simulink model "IEEE_1547_fast_function"  (Simulink 9.2)
settings: Solver=ode4  StartTime=0.0  StopTime=5  FixedStep=Ts  RelTol=1e-3  EnableMultiTasking=on
PreLoadFcn:
  | Ts=40e-6;dec=1;Tend=170;Tstart=10;Nsig=10;Nbss=500;
PostLoadFcn:
  | Ts=40e-6;dec=1;Tend=170;Tstart=10;Nsig=10;Nbss=500;
InitFcn:
  | Ts=40e-6;dec=1;Tend=170;Tstart=10;Nsig=10;Nbss=500;
undefined symbols (not defined in the file or in its folder): magnitude
libraries: simulink x15, powerlib_meascontrol x15, rtlab x3, pePowerMeasurement x3, rtio_opalrt_common x2, powerlib x1
settings Model: ARTEMISmethode_block_infos=$$__separator__$$  Creator=DETLDAQ  LastModifiedBy=apabl  NumberOfSteps=10
settings DataIOCC: SignalLoggingSaveFormat=Dataset
settings OptimizationCC: BlockReduction=off  BooleanDataType=off  OptimizeBlockIOStorage=off  BufferReuse=off  GlobalBufferReuse=off  ExpressionFolding=off  LocalBlockOutputs=off  OptimizeDataStoreBuffers=off  BusAssignmentInplaceUpdate=off
settings DebuggingCC: SaveWithParameterizedLinksMsg=none  SignalResolutionControl=TryResolveAllWithWarning  MultiTaskDSMMsg=warning  MultiTaskCondExecSysMsg=none  FcnCallInpInsideContextMsg=error
settings HardwareCC: TargetBitPerPointer=64  TargetBitPerSizeT=64  TargetBitPerPtrDiffT=64  TargetLongLongMode=on  TargetIntDivRoundTo=Zero  TargetEndianess=LittleEndian  TargetWordSize=64  TargetHWDeviceType=MATLAB Host  ProdEqTarget=off
settings GRTTargetCC: CombineOutputUpdateFcns=on  GRTInterface=off
settings SimscapeCC: SimscapeNormalizeSystem=off

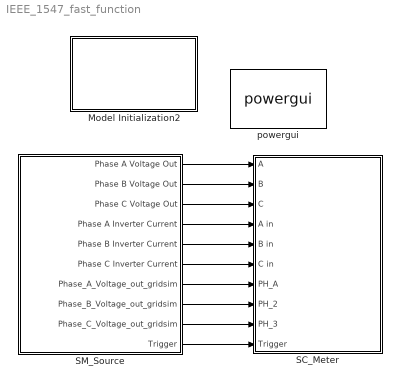
== system IEEE_1547_fast_function ==
  Model Initialization2 : Subsystem  AncestorBlock=artemis/Tools /Misc/Model Initialization  mask(Model Functions){InitFcnX=Ts=40e-6;dec=1;Tend=170;Tstart=10;Nsig=10;Nbss=500;, prel=on, posl=on, inif=on, strf=off}
      mask prompts: InitFcnX "Initialisation"; prel "Preload Function"; posl "PostLoad Function"; inif "InitFcn"; strf "StartFcn"
      mask init:
      | currentBlock = gcb;
      | root = bdroot(currentBlock);
      | 
      | if ~strcmp(get_param(root,'BlockDiagramType'),'library')
      |     if prel==1
      |         set_param(root, 'PreLoadFcn', InitFcnX);
      |     else
      |         set_param(root, 'PreLoadFcn', '');
      |     end
      |     if inif==1
      |         set_param(root, 'InitFcn', InitFcnX);
      |     else
      |         set_param(root, 'InitFcn', '');
      |     end
      |     if strf==1
      |         set_param(root, 'StartFcn', InitFcnX);
      |     else
      |         set_param(root, 'StartFcn', '');
      |     end
      |     if posl==1
      |         set_param(root, 'PostLoadFcn', InitFcnX);
      |     else
      |         set_param(root, 'PostLoadFcn', '');
      |     end
      | end
      | 
      | pos = get_param(currentBlock, 'Position');
      | width = pos(3) - pos(1); height = pos(4) - pos(2);
      | txt = [ upper(root) '\n' '- InitFcn. . . . . '  get_param(root, 'InitFcn') ];
      settings: CopyFcn=set_param(gcb,'LinkStatus','inactive')
      mask Display: text(5, height*0.5, txt, 'horizontalAlignment', 'left', 'verticalAlignment', 'middle') ;
  SC_Meter : Subsystem
  SM_Source : Subsystem
  powergui : powerlib/powergui  Priority=1  SimulationMode=Discrete  SampleTime=Ts  frequency=60  Iterations=50  frequencyindice=0  Pbase=100e6  ErrMax=1e-4  UnitsV=kV  UnitsW=MW  buscounter=0  FunctionMessages=off  echomessages=off  EnableUseOfTLC=off  CurrentSourceSwitches=off  DisableSnubberDevices=off  DisableRonSwitches=off  DisableVfSwitches=off  DisplayEquations=off  SolverType=Backward Euler  Interpol=off  ExternalGateDelay=off  methode=off  Ts=100  x0status=blocks  SPID=off  SwTol=0  HookPort=off  RestoreLinks=warning  ResistiveCurrentMeasurement=off  Frange=[0:2:500]  Ylog=off  Xlog=on  ShowGrid=off  save=off  variable=ZData  structure=0  ZoomFFT=off  StartTime=0.0  cycles=1  DisplayStyle=1  fundamental=60  FreqAxis=off  MaxFrequency=1000  frequencyindicesteady=1  RmsSteady=1  display=off
  wires:
  SM_Source/5(Phase B Inverter Current) -> SC_Meter/5(B in)
  SM_Source/6(Phase C Inverter Current) -> SC_Meter/6(C in)
  SM_Source/4(Phase A Inverter Current) -> SC_Meter/4(A in)
  SM_Source/2(Phase B Voltage Out) -> SC_Meter/2(B)
  SM_Source/1(Phase A Voltage Out) -> SC_Meter/1(A)
  SM_Source/3(Phase C Voltage Out) -> SC_Meter/3(C)
  SM_Source/7(Phase_A_Voltage_out_gridsim) -> SC_Meter/7(PH_A)
  SM_Source/8(Phase_B_Voltage_out_gridsim) -> SC_Meter/8(PH_2)
  SM_Source/9(Phase_C_Voltage_out_gridsim) -> SC_Meter/9(PH_3)
  SM_Source/10(Trigger) -> SC_Meter/10(Trigger)

== system IEEE_1547_fast_function/Model Initialization2 ==

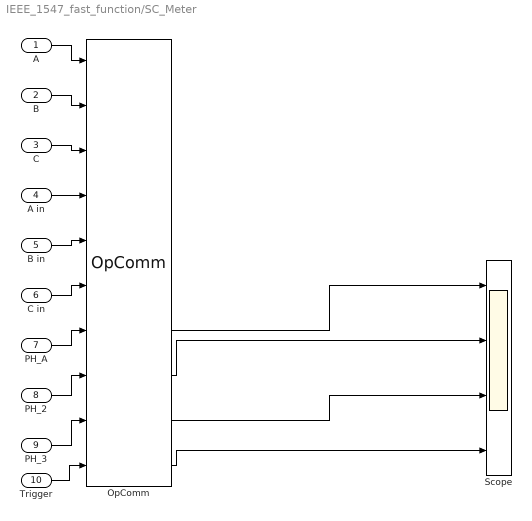
== system IEEE_1547_fast_function/SC_Meter ==
  A : Inport
  B : Inport  Port=2
  C : Inport  Port=3
  A in : Inport  Port=4
  B in : Inport  Port=5
  C in : Inport  Port=6
  PH_A : Inport  Port=7
  PH_2 : Inport  Port=8
  PH_3 : Inport  Port=9
  Trigger : Inport  Port=10
  OpComm : rtlab/OpComm  nbport=10  groupe_acq=1  subsys_rate=Ts  st=0  Synchronization=on  Interpolation=on  Threshold=1.0  Missed_Data=off  Sim_Time=off  Samples=off  dynSigOut=off  from_console=0  warning_done=off  writeOpCommFile=off  Offset=off
      settings: SourceProductName=RT-LAB
  Scope : Scope  NumInputPorts=4
  wires:
  A/1 -> OpComm/1
  B/1 -> OpComm/2
  C/1 -> OpComm/3
  A in/1 -> OpComm/4
  B in/1 -> OpComm/5
  C in/1 -> OpComm/6
  PH_A/1 -> OpComm/7
  PH_2/1 -> OpComm/8
  PH_3/1 -> OpComm/9
  Trigger/1 -> OpComm/10
  OpComm/10 -> Scope/4
  OpComm/7 -> Scope/1
  OpComm/8 -> Scope/2
  OpComm/9 -> Scope/3

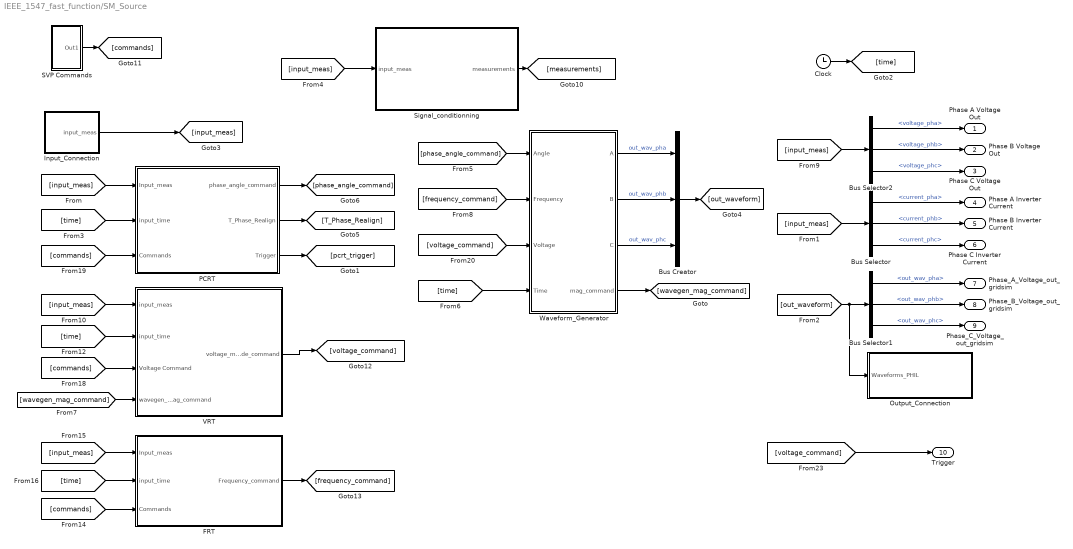
== system IEEE_1547_fast_function/SM_Source ==
  Bus Creator : BusCreator  Inputs=3
  Bus Selector : BusSelector  OutputSignals=current_pha,current_phb,current_phc
  Bus Selector1 : BusSelector  OutputSignals=out_wav_pha,out_wav_phb,out_wav_phc
  Bus Selector2 : BusSelector  OutputSignals=voltage_pha,voltage_phb,voltage_phc
  Clock : Clock
  FRT : Subsystem
  Input_Connection : Subsystem
  Output_Connection : Subsystem
  PCRT : Subsystem
  SVP Commands : Subsystem
  Signal_conditionning : Subsystem
  VRT : Subsystem
  Waveform_Generator : Subsystem
  Phase A Voltage Out : Outport
  Phase B Voltage Out : Outport  Port=2
  Phase C Voltage Out : Outport  Port=3
  Phase A Inverter Current : Outport  Port=4
  Phase B Inverter Current : Outport  Port=5
  Phase C Inverter Current : Outport  Port=6
  Phase_A_Voltage_out_gridsim : Outport  Port=7
  Phase_B_Voltage_out_gridsim : Outport  Port=8
  Phase_C_Voltage_out_gridsim : Outport  Port=9
  Trigger : Outport  Port=10
  wires:
  [frequency_command] -> Waveform_Generator/2(Frequency)
  [voltage_command] -> Waveform_Generator/3(Voltage)
  Input_Connection/1(input_meas) -> [input_meas]
  [input_meas] -> PCRT/1(Input_meas)
  [input_meas] -> Bus Selector/1
  Bus Selector/1 -> Phase A Inverter Current/1  "<current_pha>"
  Bus Selector/2 -> Phase B Inverter Current/1  "<current_phb>"
  Bus Selector/3 -> Phase C Inverter Current/1  "<current_phc>"
  Waveform_Generator/1(A) -> Bus Creator/1  "out_wav_pha"
  Waveform_Generator/2(B) -> Bus Creator/2  "out_wav_phb"
  Waveform_Generator/3(C) -> Bus Creator/3  "out_wav_phc"
  Bus Creator/1 -> [out_waveform]
  Bus Selector1/2 -> Phase_B_Voltage_out_gridsim/1  "<out_wav_phb>"
  Bus Selector1/1 -> Phase_A_Voltage_out_gridsim/1  "<out_wav_pha>"
  [out_waveform] -> Output_Connection/1(Waveforms_PHIL), Bus Selector1/1
  Bus Selector1/3 -> Phase_C_Voltage_out_gridsim/1  "<out_wav_phc>"
  PCRT/3(Trigger) -> [pcrt_trigger]
  Clock/1 -> [time]
  [time] -> PCRT/2(input_time)
  [input_meas] -> Signal_conditionning/1(input_meas)
  Signal_conditionning/1(measurements) -> [measurements]
  PCRT/2(T_Phase_Realign) -> [T_Phase_Realign]
  PCRT/1(phase_angle_command) -> [phase_angle_command]
  [phase_angle_command] -> Waveform_Generator/1(Angle)
  Bus Selector2/2 -> Phase B Voltage Out/1  "<voltage_phb>"
  Bus Selector2/1 -> Phase A Voltage Out/1  "<voltage_pha>"
  [input_meas] -> Bus Selector2/1
  Bus Selector2/3 -> Phase C Voltage Out/1  "<voltage_phc>"
  [voltage_command] -> Trigger/1
  [time] -> VRT/2(input_time)
  [input_meas] -> VRT/1(input_meas)
  [time] -> FRT/2(input_time)
  [input_meas] -> FRT/1(Input_meas)
  SVP Commands/1(Out1) -> [commands]
  [commands] -> VRT/3(Voltage Command)
  [commands] -> PCRT/3(Commands)
  VRT/1(voltage_magnitude_command) -> [voltage_command]
  [commands] -> FRT/3(Commands)
  FRT/1(Frequency_command) -> [frequency_command]
  [time] -> Waveform_Generator/4(Time)
  Waveform_Generator/4(mag_command) -> [wavegen_mag_command]
  [wavegen_mag_command] -> VRT/4(wavegen_mag_command)

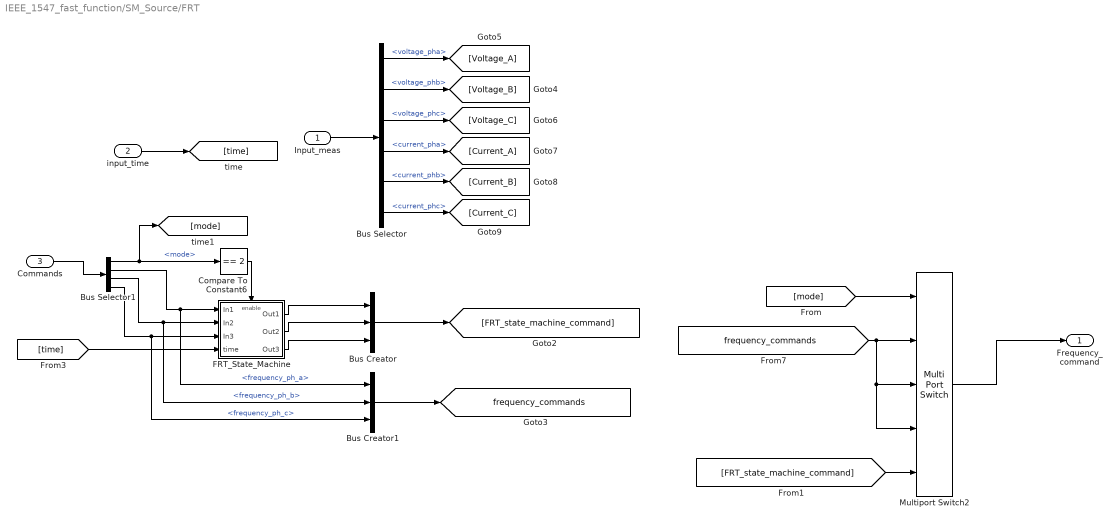
== system IEEE_1547_fast_function/SM_Source/FRT ==
  Input_meas : Inport
  input_time : Inport  Port=2
  Commands : Inport  Port=3
  Bus Creator : BusCreator  Inputs=3
  Bus Creator1 : BusCreator  Inputs=3
  Bus Selector : BusSelector  OutputSignals=voltage_pha,voltage_phb,voltage_phc,current_pha,current_phb,current_phc
  Bus Selector1 : BusSelector  OutputSignals=mode,frequency_ph_a,frequency_ph_b,frequency_ph_c
  Compare To Constant6 : simulink/Logic and Bit Operations/Compare To Constant  relop===  const=2  OutDataTypeStr=boolean
  FRT_State_Machine : Subsystem
  Multiport Switch2 : MultiPortSwitch  Inputs=4
  Frequency_command : Outport
  tag scope: frequency_commands=global
  wires:
  Input_meas/1 -> Bus Selector/1
  input_time/1 -> [time]
  FRT_State_Machine/1(Out1) -> Bus Creator/1
  FRT_State_Machine/2(Out2) -> Bus Creator/2
  FRT_State_Machine/3(Out3) -> Bus Creator/3
  Compare To Constant6/1 -> FRT_State_Machine/Enable
  Multiport Switch2/1 -> Frequency_command/1
  [mode] -> Multiport Switch2/1
  Bus Creator/1 -> [FRT_state_machine_command]
  Bus Creator1/1 -> [frequency_commands]
  [time] -> FRT_State_Machine/4(time)
  Bus Selector/1 -> [Voltage_A]  "<voltage_pha>"
  Bus Selector/2 -> [Voltage_B]  "<voltage_phb>"
  Bus Selector/3 -> [Voltage_C]  "<voltage_phc>"
  Bus Selector/4 -> [Current_A]  "<current_pha>"
  Bus Selector/5 -> [Current_B]  "<current_phb>"
  Bus Selector/6 -> [Current_C]  "<current_phc>"
  [FRT_state_machine_command] -> Multiport Switch2/5
  Commands/1 -> Bus Selector1/1
  Bus Selector1/1 -> [mode], Compare To Constant6/1  "<mode>"
  Bus Selector1/2 -> Bus Creator1/1, FRT_State_Machine/1(In1)  "<frequency_ph_a>"
  Bus Selector1/3 -> Bus Creator1/2, FRT_State_Machine/2(In2)  "<frequency_ph_b>"
  Bus Selector1/4 -> Bus Creator1/3, FRT_State_Machine/3(In3)  "<frequency_ph_c>"
  [frequency_commands] -> Multiport Switch2/3, Multiport Switch2/4, Multiport Switch2/2

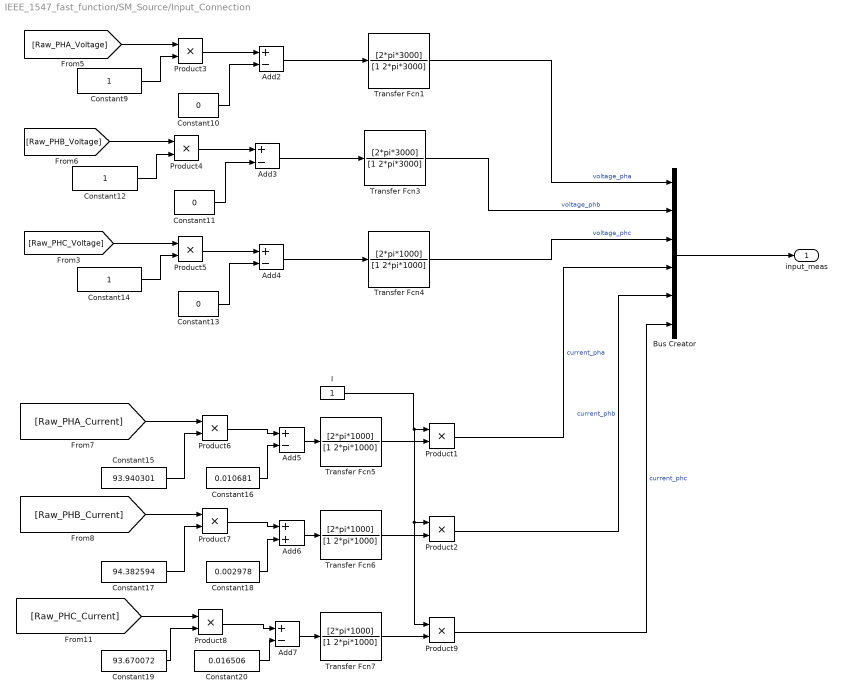
== system IEEE_1547_fast_function/SM_Source/Input_Connection ==
  Add{2..5,7} (5 alike) : Sum  Inputs=+-
  Add6 : Sum
  Bus Creator : BusCreator  Inputs=6
  Constant10 : Constant  Value=0
  Constant11 : Constant  Value=0
  Constant12 : Constant
  Constant13 : Constant  Value=0
  Constant14 : Constant
  Constant15 : Constant  Value=93.940301
  Constant16 : Constant  Value=0.010681
  Constant17 : Constant  Value=94.382594
  Constant18 : Constant  Value=0.002978
  Constant19 : Constant  Value=93.670072
  Constant20 : Constant  Value=0.016506
  Constant9 : Constant
  I : Constant
  Product{1..9} (9 alike) : Product
  Transfer Fcn1 : TransferFcn  Numerator=[2*pi*3000]  Denominator=[1 2*pi*3000]
  Transfer Fcn3 : TransferFcn  Numerator=[2*pi*3000]  Denominator=[1 2*pi*3000]
  Transfer Fcn{4..7} (4 alike) : TransferFcn  Numerator=[2*pi*1000]  Denominator=[1 2*pi*1000]
  input_meas : Outport
  wires:
  [Raw_PHB_Current] -> Product7/1
  Product6/1 -> Add5/1
  Add3/1 -> Transfer Fcn3/1
  Constant17/1 -> Product7/2
  I/1 -> Product9/1, Product2/1, Product1/1
  Transfer Fcn6/1 -> Product2/2
  Constant14/1 -> Product5/2
  Constant10/1 -> Add2/2
  Add4/1 -> Transfer Fcn4/1
  Constant13/1 -> Add4/2
  [Raw_PHB_Voltage] -> Product4/1
  Product8/1 -> Add7/1
  Product5/1 -> Add4/1
  Constant15/1 -> Product6/2
  [Raw_PHC_Voltage] -> Product5/1
  Constant20/1 -> Add7/2
  Add6/1 -> Transfer Fcn6/1
  Add5/1 -> Transfer Fcn5/1
  Product7/1 -> Add6/1
  Add2/1 -> Transfer Fcn1/1
  [Raw_PHA_Voltage] -> Product3/1
  Constant18/1 -> Add6/2
  [Raw_PHA_Current] -> Product6/1
  Transfer Fcn7/1 -> Product9/2
  [Raw_PHC_Current] -> Product8/1
  Add7/1 -> Transfer Fcn7/1
  Constant16/1 -> Add5/2
  Transfer Fcn5/1 -> Product1/2
  Constant9/1 -> Product3/2
  Constant12/1 -> Product4/2
  Product4/1 -> Add3/1
  Constant11/1 -> Add3/2
  Product3/1 -> Add2/1
  Constant19/1 -> Product8/2
  Transfer Fcn1/1 -> Bus Creator/1  "voltage_pha"
  Transfer Fcn3/1 -> Bus Creator/2  "voltage_phb"
  Transfer Fcn4/1 -> Bus Creator/3  "voltage_phc"
  Product1/1 -> Bus Creator/4  "current_pha"
  Product2/1 -> Bus Creator/5  "current_phb"
  Product9/1 -> Bus Creator/6  "current_phc"
  Bus Creator/1 -> input_meas/1

== system IEEE_1547_fast_function/SM_Source/Output_Connection ==
  Waveforms_PHIL : Inport
  AnalogOut : rtio_opalrt_common/AnalogOut  CtrlName='OpCtrl'  portNb=19  FcnNos=Slot 1 Module A Subsection 1  size=32  maxcount=-2  count=8  numchan=8  israngeinput=off  voltagerange=[-16 ... 16]  slot=0  side=0  mismatch=0  slotside=Slot_1_Module_A
      settings: AttributesFormatString=%<CtrlName>
  Bus Selector : BusSelector  OutputSignals=out_wav_pha,out_wav_phb,out_wav_phc
  Mux1 : Mux  Inputs=8
  OpCtrl : rtio_opalrt_common/OpCtrl  CtrlName='OpCtrl'  boardid=0  BitstreamFilename=VC707_2-EX-0001-3_1_6_559-eHSx128_2xC3C1FBCD-35-18.bin  numconfig=-1  mode=Master  externalClock=off  decimRtsi=0  calibIO=off  SampleTime=0  loadinport=-1  BoardType=VC707  SecondaryPresent=off  sync_type=Optical fiber  scope_enable=off  scope_acqPeriodSec=0  scope_trigPos=0
  Terminator : Terminator
  out_wav_pha : Gain
  out_wav_phb : Gain
  out_wav_phc : Gain
  wires:
  Mux1/1 -> AnalogOut/1
  AnalogOut/1 -> Terminator/1
  Waveforms_PHIL/1 -> Bus Selector/1
  Bus Selector/2 -> out_wav_phb/1  "<out_wav_phb>"
  Bus Selector/3 -> out_wav_phc/1  "<out_wav_phc>"
  Bus Selector/1 -> out_wav_pha/1  "<out_wav_pha>"
  out_wav_pha/1 -> Mux1/1
  out_wav_phb/1 -> Mux1/2
  out_wav_phc/1 -> Mux1/4

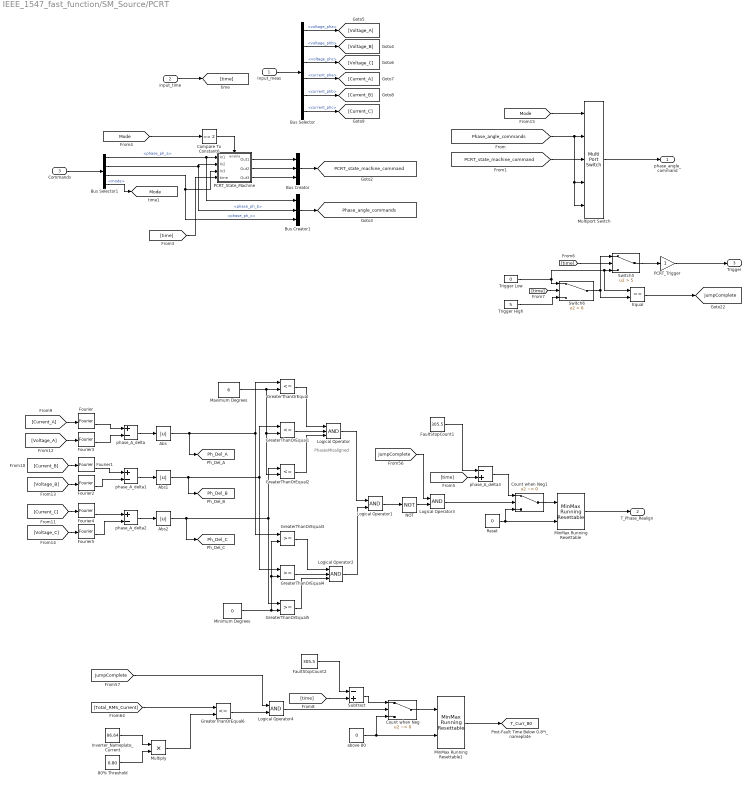
== system IEEE_1547_fast_function/SM_Source/PCRT ==
  note: PhasesMisaligned
  Input_meas : Inport
  input_time : Inport  Port=2
  Commands : Inport  Port=3
  80% Threshold : Constant  Value=0.80
  Abs : Abs
  Abs1 : Abs
  Abs2 : Abs
  Bus Creator : BusCreator  Inputs=3
  Bus Creator1 : BusCreator  Inputs=3
  Bus Selector : BusSelector  OutputSignals=voltage_pha,voltage_phb,voltage_phc,current_pha,current_phb,current_phc
  Bus Selector1 : BusSelector  OutputSignals=phase_ph_a,phase_ph_b,phase_ph_c,mode
  Compare To Constant6 : simulink/Logic and Bit Operations/Compare To Constant  relop===  const=2  OutDataTypeStr=boolean
  Count when Neg : Switch  Criteria=u2 ~= 0
  Count when Neg1 : Switch  Criteria=u2 ~= 0
  Equal : RelationalOperator  Operator===  OutDataTypeStr=boolean  RndMeth=Simplest
  FaultStopCount1 : Constant  Value=305.5
  FaultStopCount2 : Constant  Value=305.5
  Fourier{,1..5} (6 alike) : powerlib_meascontrol/Measurements/Fourier  Freq=60  n=1  InInit=[0, 0]  Ts=0
      settings: SourceProductName=Simscape Power Systems
  GreaterThanOrEqual{,1..2,6} (4 alike) : RelationalOperator  Operator=<=  OutDataTypeStr=boolean  RndMeth=Simplest
  GreaterThanOrEqual3 : RelationalOperator  OutDataTypeStr=boolean  RndMeth=Simplest
  GreaterThanOrEqual4 : RelationalOperator  OutDataTypeStr=boolean  RndMeth=Simplest
  GreaterThanOrEqual5 : RelationalOperator  OutDataTypeStr=boolean  RndMeth=Simplest
  Inverter_Nameplate_Current : Constant  Value=86.64
  Logical Operator : Logic  Inputs=3  AllPortsSameDT=off  OutDataTypeStr=boolean
  Logical Operator1 : Logic  AllPortsSameDT=off  OutDataTypeStr=boolean
  Logical Operator2 : Logic  Inputs=3  AllPortsSameDT=off  OutDataTypeStr=boolean
  Logical Operator3 : Logic  AllPortsSameDT=off  OutDataTypeStr=boolean
  Logical Operator4 : Logic  AllPortsSameDT=off  OutDataTypeStr=boolean
  Maximum Degrees : Constant  Value=6
  MinMax Running Resettable : simulink/Math Operations/MinMax Running Resettable  Function=max  vinit=0.0
  MinMax Running Resettable1 : simulink/Math Operations/MinMax Running Resettable  Function=max  vinit=0.0
  Minimum Degrees : Constant  Value=0
  Multiply : Product
  Multiport Switch : MultiPortSwitch  Inputs=4
  NOT : Logic  Operator=NOT  IconShape=distinctive  AllPortsSameDT=off  OutDataTypeStr=boolean
  PCRT_State_Machine : Subsystem
  PCRT_Trigger : Gain
  Reset : Constant  Value=0
  Subtract : Sum  Inputs=-+
  Switch5 : Switch  Criteria=u2 > Threshold  Threshold=5
  Switch6 : Switch  Criteria=u2 > Threshold  Threshold=6
  Trigger High : Constant  Value=5
  Trigger Low : Constant  Value=0
  above 80 : Constant  Value=0
  phase_A_delta : Sum  Inputs=+-
  phase_A_delta1 : Sum  Inputs=+-
  phase_A_delta2 : Sum  Inputs=+-
  phase_A_delta3 : Sum  Inputs=-+
  phase_angle_command : Outport
  T_Phase_Realign : Outport  Port=2
  Trigger : Outport  Port=3
  tag scope: JumpComplete=global, Mode=global, PCRT_state_machine_command=global, Ph_Del_A=global, Ph_Del_B=global, Ph_Del_C=global, Phase_angle_commands=global, T_Curr_80=global
  wires:
  Abs/1 -> GreaterThanOrEqual/1, GreaterThanOrEqual3/1, [Ph_Del_A]
  Abs2/1 -> GreaterThanOrEqual2/1, GreaterThanOrEqual5/1, [Ph_Del_C]
  phase_A_delta2/1 -> Abs2/1
  Abs1/1 -> GreaterThanOrEqual1/1, GreaterThanOrEqual4/1, [Ph_Del_B]
  GreaterThanOrEqual5/1 -> Logical Operator2/3
  Minimum Degrees/1 -> GreaterThanOrEqual3/2, GreaterThanOrEqual4/2, GreaterThanOrEqual5/2
  GreaterThanOrEqual/1 -> Logical Operator/1
  Reset/1 -> MinMax Running Resettable/2, Count when Neg1/3
  GreaterThanOrEqual4/1 -> Logical Operator2/2
  GreaterThanOrEqual3/1 -> Logical Operator2/1
  Logical Operator3/1 -> Count when Neg1/2
  NOT/1 -> Logical Operator3/2
  Logical Operator/1 -> Logical Operator1/1
  Fourier3/2 -> phase_A_delta/2
  Logical Operator2/1 -> Logical Operator1/2
  Logical Operator1/1 -> NOT/1
  GreaterThanOrEqual1/1 -> Logical Operator/2
  [time] -> phase_A_delta3/2
  FaultStopCount1/1 -> phase_A_delta3/1
  Maximum Degrees/1 -> GreaterThanOrEqual/2, GreaterThanOrEqual2/2, GreaterThanOrEqual1/2
  MinMax Running Resettable/1 -> T_Phase_Realign/1
  [JumpComplete] -> Logical Operator3/1
  phase_A_delta3/1 -> Count when Neg1/1
  phase_A_delta/1 -> Abs/1
  Fourier/2 -> phase_A_delta/1
  Count when Neg1/1 -> MinMax Running Resettable/1
  Fourier5/2 -> phase_A_delta2/2
  phase_A_delta1/1 -> Abs1/1
  Fourier4/2 -> phase_A_delta2/1
  GreaterThanOrEqual2/1 -> Logical Operator/3
  Fourier1/2 -> phase_A_delta1/1
  Fourier2/2 -> phase_A_delta1/2
  Input_meas/1 -> Bus Selector/1
  Trigger High/1 -> Switch6/3
  Equal/1 -> [JumpComplete]
  [time] -> Switch6/2
  Trigger Low/1 -> Equal/1, Switch5/3, Switch6/1
  PCRT_Trigger/1 -> Trigger/1
  Switch6/1 -> Equal/2, Switch5/1
  [time] -> Switch5/2
  Switch5/1 -> PCRT_Trigger/1
  input_time/1 -> [time]
  [time] -> Subtract/2
  FaultStopCount2/1 -> Subtract/1
  [JumpComplete] -> Logical Operator4/1
  Subtract/1 -> Count when Neg/1
  Multiply/1 -> GreaterThanOrEqual6/2
  Count when Neg/1 -> MinMax Running Resettable1/1
  above 80/1 -> Count when Neg/3, MinMax Running Resettable1/2
  Inverter_Nameplate_Current/1 -> Multiply/1
  [Total_RMS_Current] -> GreaterThanOrEqual6/1
  Logical Operator4/1 -> Count when Neg/2
  GreaterThanOrEqual6/1 -> Logical Operator4/2
  MinMax Running Resettable1/1 -> [T_Curr_80]
  80% Threshold/1 -> Multiply/2
  Bus Selector1/2 -> Bus Creator1/2, PCRT_State_Machine/2(In2)  "<phase_ph_b>"
  Bus Selector1/3 -> Bus Creator1/3, PCRT_State_Machine/3(In3)  "<phase_ph_c>"
  PCRT_State_Machine/1(Out1) -> Bus Creator/1
  PCRT_State_Machine/2(Out2) -> Bus Creator/2
  PCRT_State_Machine/3(Out3) -> Bus Creator/3
  Compare To Constant6/1 -> PCRT_State_Machine/Enable
  Multiport Switch/1 -> phase_angle_command/1
  [Mode] -> Multiport Switch/1
  Bus Creator/1 -> [PCRT_state_machine_command]
  Bus Creator1/1 -> [Phase_angle_commands]
  [time] -> PCRT_State_Machine/4(time)
  [Mode] -> Compare To Constant6/1
  Bus Selector/1 -> [Voltage_A]  "<voltage_pha>"
  Bus Selector/2 -> [Voltage_B]  "<voltage_phb>"
  Bus Selector/3 -> [Voltage_C]  "<voltage_phc>"
  Bus Selector/4 -> [Current_A]  "<current_pha>"
  Bus Selector/5 -> [Current_B]  "<current_phb>"
  Bus Selector/6 -> [Current_C]  "<current_phc>"
  [Current_A] -> Fourier/1
  [Current_C] -> Fourier4/1
  [Current_B] -> Fourier1/1
  [Voltage_A] -> Fourier3/1
  [Voltage_B] -> Fourier2/1
  [Voltage_C] -> Fourier5/1
  Commands/1 -> Bus Selector1/1
  Bus Selector1/1 -> Bus Creator1/1, PCRT_State_Machine/1(In1)  "<phase_ph_a>"
  Bus Selector1/4 -> [Mode]  "<mode>"
  [PCRT_state_machine_command] -> Multiport Switch/3
  [Phase_angle_commands] -> Multiport Switch/5, Multiport Switch/4, Multiport Switch/2

== system IEEE_1547_fast_function/SM_Source/SVP Commands ==
  note: Mode :
      |
      | Nothing
      | 1
      |
      | PCRT
      | 2
      |
      | VRT
      | 3
      |
      | FRT
      | 4
  Bus Creator : BusCreator  Inputs=10
  frequency_ph_a : Constant  Value=60
  frequency_ph_b : Constant  Value=60
  frequency_ph_c : Constant  Value=60
  mode : Constant  Value=3
  phase_ph_a : Constant  Value=0
  phase_ph_b : Constant  Value=-120
  phase_ph_c : Constant  Value=120
  voltage_ph_a : Constant
  voltage_ph_b : Constant
  voltage_ph_c : Constant
  Out1 : Outport
  wires:
  phase_ph_b/1 -> Bus Creator/2  "phase_ph_b"
  phase_ph_c/1 -> Bus Creator/3  "phase_ph_c"
  phase_ph_a/1 -> Bus Creator/1  "phase_ph_a"
  voltage_ph_a/1 -> Bus Creator/4  "voltage_ph_a"
  voltage_ph_c/1 -> Bus Creator/6  "voltage_ph_c"
  voltage_ph_b/1 -> Bus Creator/5  "voltage_ph_b"
  frequency_ph_b/1 -> Bus Creator/8  "frequency_ph_b"
  frequency_ph_c/1 -> Bus Creator/9  "frequency_ph_c"
  frequency_ph_a/1 -> Bus Creator/7  "frequency_ph_a"
  mode/1 -> Bus Creator/10  "mode"
  Bus Creator/1 -> Out1/1

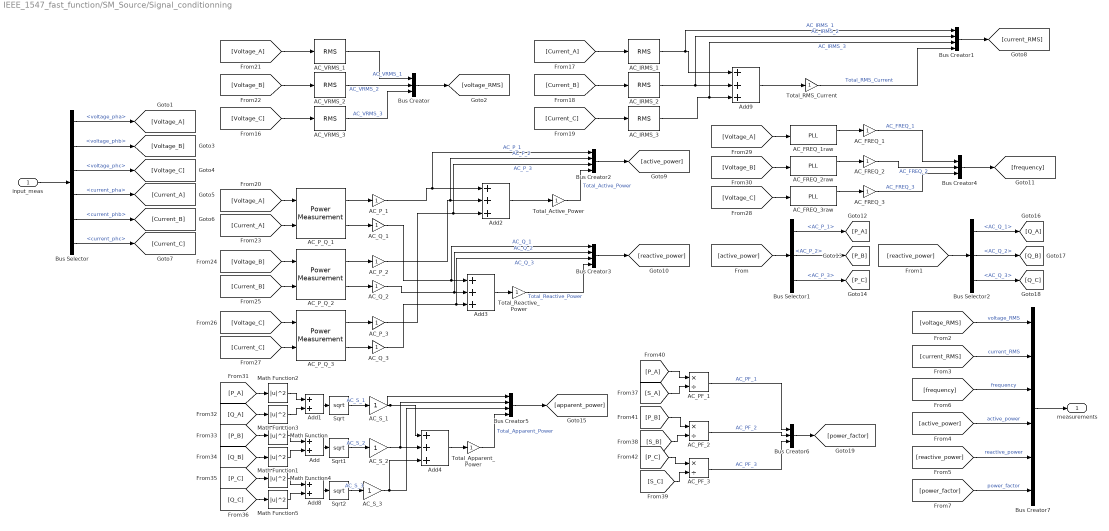
== system IEEE_1547_fast_function/SM_Source/Signal_conditionning ==
  input_meas : Inport
  AC_FREQ_1 : Gain
  AC_FREQ_1raw : powerlib_meascontrol/PLL/PLL  Fmin=45  Par_Init=[0, 60]  ParK=[180, 3200, 1]  TcD=1e-4  MaxRateChangeFreq=12  FilterCutOffFreq=25  Ts=0  AGC=on
      settings: SourceProductName=Simscape Power Systems  SourceProductBaseCode=PS
  AC_FREQ_2 : Gain
  AC_FREQ_2raw : powerlib_meascontrol/PLL/PLL  Fmin=45  Par_Init=[0, 60]  ParK=[180, 3200, 1]  TcD=1e-4  MaxRateChangeFreq=12  FilterCutOffFreq=25  Ts=0  AGC=on
      settings: SourceProductName=Simscape Power Systems  SourceProductBaseCode=PS
  AC_FREQ_3 : Gain
  AC_FREQ_3raw : powerlib_meascontrol/PLL/PLL  Fmin=45  Par_Init=[0, 60]  ParK=[180, 3200, 1]  TcD=1e-4  MaxRateChangeFreq=12  FilterCutOffFreq=25  Ts=0  AGC=on
      settings: SourceProductName=Simscape Power Systems  SourceProductBaseCode=PS
  AC_IRMS_1 : powerlib_meascontrol/Measurements/RMS  TrueRMS=on  Freq=60  RMSInit=120  Ts=0
  AC_IRMS_2 : powerlib_meascontrol/Measurements/RMS  TrueRMS=on  Freq=60  RMSInit=120  Ts=0
  AC_IRMS_3 : powerlib_meascontrol/Measurements/RMS  TrueRMS=on  Freq=60  RMSInit=120  Ts=0
  AC_PF_1 : Product  Inputs=*/
  AC_PF_2 : Product  Inputs=*/
  AC_PF_3 : Product  Inputs=*/
  AC_P_1 : Gain
  AC_P_2 : Gain
  AC_P_3 : Gain
  AC_P_Q_1 : pePowerMeasurement/Power Measurement  LabelModeActiveChoice=Continuous  F=60  K=[0 1 2 3]  Ts=0
  AC_P_Q_2 : pePowerMeasurement/Power Measurement  LabelModeActiveChoice=Continuous  F=60  K=[0 1 2 3]  Ts=0
  AC_P_Q_3 : pePowerMeasurement/Power Measurement  LabelModeActiveChoice=Continuous  F=60  K=[0 1 2 3]  Ts=0
  AC_Q_1 : Gain
  AC_Q_2 : Gain
  AC_Q_3 : Gain
  AC_S_1 : Gain
  AC_S_2 : Gain
  AC_S_3 : Gain
  AC_VRMS_1 : powerlib_meascontrol/Measurements/RMS  TrueRMS=on  Freq=60  RMSInit=120  Ts=0
  AC_VRMS_2 : powerlib_meascontrol/Measurements/RMS  TrueRMS=on  Freq=60  RMSInit=120  Ts=0
  AC_VRMS_3 : powerlib_meascontrol/Measurements/RMS  TrueRMS=on  Freq=60  RMSInit=120  Ts=0
  Add : Sum
  Add1 : Sum
  Add{2..4,9} (4 alike) : Sum  Inputs=+++
  Add8 : Sum
  Bus Creator : BusCreator  Inputs=3
  Bus Creator{1..3,5} (4 alike) : BusCreator  Inputs=4
  Bus Creator4 : BusCreator  Inputs=3
  Bus Creator6 : BusCreator  Inputs=3
  Bus Creator7 : BusCreator  Inputs=6
  Bus Selector : BusSelector  OutputSignals=voltage_pha,voltage_phb,voltage_phc,current_pha,current_phb,current_phc
  Bus Selector1 : BusSelector  OutputSignals=AC_P_1,AC_P_2,AC_P_3
  Bus Selector2 : BusSelector  OutputSignals=AC_Q_1,AC_Q_2,AC_Q_3
  Math Function{,1..5} (6 alike) : Math  Operator=magnitude^2  SaturateOnIntegerOverflow=on
  Sqrt : Sqrt  SaturateOnIntegerOverflow=on
  Sqrt1 : Sqrt  SaturateOnIntegerOverflow=on
  Sqrt2 : Sqrt  SaturateOnIntegerOverflow=on
  Total_Active_Power : Gain
  Total_Apparent_Power : Gain
  Total_RMS_Current : Gain
  Total_Reactive_Power : Gain
  measurements : Outport
  wires:
  [Current_B] -> AC_IRMS_2/1
  [P_A] -> AC_PF_1/1
  Math Function4/1 -> Add8/1
  [Voltage_A] -> AC_P_Q_1/1
  [Current_C] -> AC_IRMS_3/1
  [Current_A] -> AC_P_Q_1/2
  [Voltage_C] -> AC_VRMS_3/1
  Sqrt1/1 -> AC_S_2/1  "AC_S_2"
  [Voltage_B] -> AC_VRMS_2/1
  Math Function1/1 -> Add/2
  AC_P_Q_1/2 -> AC_Q_1/1
  Math Function5/1 -> Add8/2
  [Voltage_B] -> AC_P_Q_2/1
  [Current_A] -> AC_IRMS_1/1
  AC_P_Q_1/1 -> AC_P_1/1
  [Voltage_C] -> AC_P_Q_3/1
  AC_P_Q_2/2 -> AC_Q_2/1
  Add8/1 -> Sqrt2/1
  AC_P_Q_3/1 -> AC_P_3/1
  [Current_B] -> AC_P_Q_2/2
  [Voltage_A] -> AC_FREQ_1raw/1
  [Q_B] -> Math Function1/1
  [Voltage_C] -> AC_FREQ_3raw/1
  [P_C] -> AC_PF_3/1
  AC_FREQ_1raw/1 -> AC_FREQ_1/1
  [S_C] -> AC_PF_3/2
  [P_B] -> Math Function/1
  AC_FREQ_2raw/1 -> AC_FREQ_2/1
  [P_B] -> AC_PF_2/1
  [Q_A] -> Math Function3/1
  [Voltage_B] -> AC_FREQ_2raw/1
  Sqrt/1 -> AC_S_1/1  "AC_S_1"
  Sqrt2/1 -> AC_S_3/1  "AC_S_3"
  [P_A] -> Math Function2/1
  Add9/1 -> Total_RMS_Current/1
  Math Function3/1 -> Add1/2
  Add1/1 -> Sqrt/1
  Math Function/1 -> Add/1
  [S_B] -> AC_PF_2/2
  [Voltage_A] -> AC_VRMS_1/1
  AC_P_Q_3/2 -> AC_Q_3/1
  Math Function2/1 -> Add1/1
  [Current_C] -> AC_P_Q_3/2
  [P_C] -> Math Function4/1
  [Q_C] -> Math Function5/1
  Add/1 -> Sqrt1/1
  AC_FREQ_3raw/1 -> AC_FREQ_3/1
  AC_P_Q_2/1 -> AC_P_2/1
  [S_A] -> AC_PF_1/2
  input_meas/1 -> Bus Selector/1
  Bus Selector/1 -> [Voltage_A]  "<voltage_pha>"
  Bus Selector/2 -> [Voltage_B]  "<voltage_phb>"
  Bus Selector/3 -> [Voltage_C]  "<voltage_phc>"
  Bus Selector/4 -> [Current_A]  "<current_pha>"
  Bus Selector/5 -> [Current_B]  "<current_phb>"
  Bus Selector/6 -> [Current_C]  "<current_phc>"
  AC_P_1/1 -> Bus Creator2/1, Add2/1  "AC_P_1"
  AC_P_2/1 -> Bus Creator2/2, Add2/2  "AC_P_2"
  AC_P_3/1 -> Bus Creator2/3, Add2/3  "AC_P_3"
  Add2/1 -> Total_Active_Power/1
  AC_Q_1/1 -> Bus Creator3/1, Add3/1  "AC_Q_1"
  AC_Q_2/1 -> Bus Creator3/2, Add3/2  "AC_Q_2"
  AC_Q_3/1 -> Bus Creator3/3, Add3/3  "AC_Q_3"
  Add3/1 -> Total_Reactive_Power/1
  Add4/1 -> Total_Apparent_Power/1
  AC_VRMS_1/1 -> Bus Creator/1  "AC_VRMS_1"
  AC_VRMS_2/1 -> Bus Creator/2  "AC_VRMS_2"
  AC_VRMS_3/1 -> Bus Creator/3  "AC_VRMS_3"
  Bus Creator/1 -> [voltage_RMS]
  AC_IRMS_1/1 -> Bus Creator1/1, Add9/1  "AC_IRMS_1"
  AC_IRMS_2/1 -> Bus Creator1/2, Add9/2  "AC_IRMS_2"
  Bus Creator1/1 -> [current_RMS]
  AC_IRMS_3/1 -> Bus Creator1/3, Add9/3  "AC_IRMS_3"
  Total_RMS_Current/1 -> Bus Creator1/4  "Total_RMS_Current"
  Total_Active_Power/1 -> Bus Creator2/4  "Total_Active_Power"
  Bus Creator2/1 -> [active_power]
  Bus Creator3/1 -> [reactive_power]
  Total_Reactive_Power/1 -> Bus Creator3/4  "Total_Reactive_Power"
  Bus Creator4/1 -> [frequency]
  AC_FREQ_1/1 -> Bus Creator4/1  "AC_FREQ_1"
  AC_FREQ_2/1 -> Bus Creator4/2  "AC_FREQ_2"
  AC_FREQ_3/1 -> Bus Creator4/3  "AC_FREQ_3"
  [active_power] -> Bus Selector1/1
  Bus Selector1/1 -> [P_A]  "<AC_P_1>"
  Bus Selector1/2 -> [P_B]  "<AC_P_2>"
  Bus Selector1/3 -> [P_C]  "<AC_P_3>"
  [reactive_power] -> Bus Selector2/1
  Bus Creator5/1 -> [apparent_power]
  Total_Apparent_Power/1 -> Bus Creator5/4  "Total_Apparent_Power"
  Bus Selector2/1 -> [Q_A]  "<AC_Q_1>"
  Bus Selector2/2 -> [Q_B]  "<AC_Q_2>"
  Bus Selector2/3 -> [Q_C]  "<AC_Q_3>"
  Bus Creator6/1 -> [power_factor]
  AC_PF_3/1 -> Bus Creator6/3  "AC_PF_3"
  AC_PF_1/1 -> Bus Creator6/1  "AC_PF_1"
  AC_PF_2/1 -> Bus Creator6/2  "AC_PF_2"
  [voltage_RMS] -> Bus Creator7/1  "voltage_RMS"
  [current_RMS] -> Bus Creator7/2  "current_RMS"
  [frequency] -> Bus Creator7/3  "frequency"
  [active_power] -> Bus Creator7/4  "active_power"
  [reactive_power] -> Bus Creator7/5  "reactive_power"
  [power_factor] -> Bus Creator7/6  "power_factor"
  Bus Creator7/1 -> measurements/1
  AC_S_1/1 -> Bus Creator5/1, Add4/1
  AC_S_2/1 -> Bus Creator5/2, Add4/2
  AC_S_3/1 -> Bus Creator5/3, Add4/3

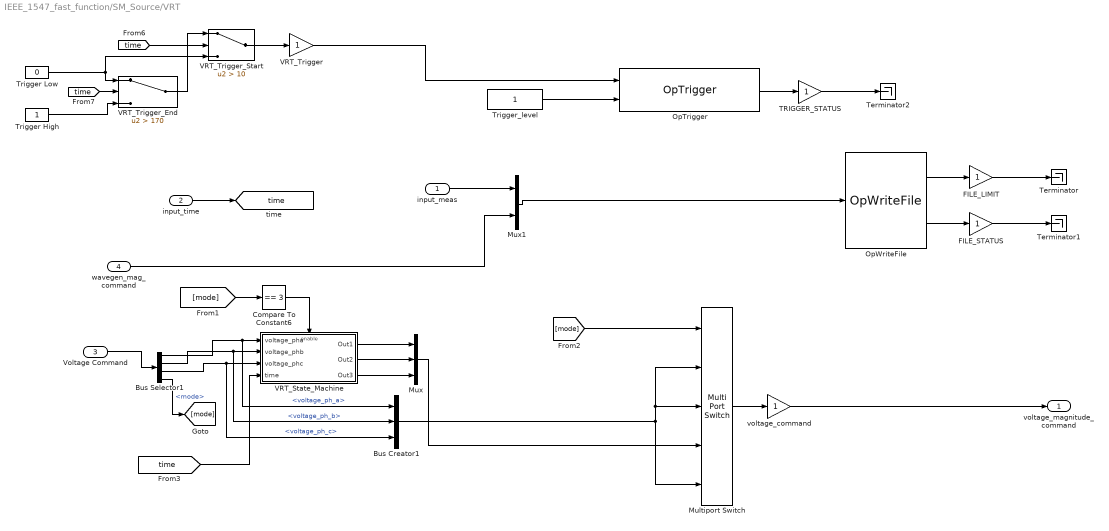
== system IEEE_1547_fast_function/SM_Source/VRT ==
  input_meas : Inport
  input_time : Inport  Port=2
  Voltage Command : Inport  Port=3
  wavegen_mag_command : Inport  Port=4
  Bus Creator1 : BusCreator  Inputs=3
  Bus Selector1 : BusSelector  OutputSignals=voltage_ph_a,voltage_ph_b,voltage_ph_c,mode
  Compare To Constant6 : simulink/Logic and Bit Operations/Compare To Constant  relop===  const=3  OutDataTypeStr=uint8
  FILE_LIMIT : Gain
  FILE_STATUS : Gain
  Multiport Switch : MultiPortSwitch  Inputs=4
  Mux : Mux  Inputs=3
  Mux1 : Mux  Inputs=2
  OpTrigger : rtlab/DataLogging/OpTrigger  Trig_Type=TRIGGER SIGNAL >= TRIGGER LEVEL  Trig_Offset=0  Acq_Group=26
      settings: SourceProductName=RT-LAB
  OpWriteFile : rtlab/DataLogging/OpWriteFile  Static_File=on  varname=Data  Filename=VRT_Data.mat  rtpath='./'  nrtpath='.\'  Acq_Group=26  file_size=2e+9  write_offline=off  Sim_Mode=off  Nb_Samples=1000  Buffer_size=88000000
      settings: SourceProductName=RT-LAB  Decimation=5
  TRIGGER_STATUS : Gain
  Terminator : Terminator
  Terminator1 : Terminator
  Terminator2 : Terminator
  Trigger High : Constant
  Trigger Low : Constant  Value=0
  Trigger_level : Constant
  VRT_State_Machine : Subsystem
  VRT_Trigger : Gain
  VRT_Trigger_End : Switch  Criteria=u2 > Threshold  Threshold=170
  VRT_Trigger_Start : Switch  Criteria=u2 > Threshold  Threshold=10
  voltage_command : Gain
  voltage_magnitude_command : Outport
  tag scope: time=global
  wires:
  [mode] -> Compare To Constant6/1
  [time] -> VRT_State_Machine/4(time)
  [mode] -> Multiport Switch/1
  Bus Creator1/1 -> Multiport Switch/2, Multiport Switch/3, Multiport Switch/5
  Compare To Constant6/1 -> VRT_State_Machine/Enable
  VRT_State_Machine/3(Out3) -> Mux/3
  VRT_State_Machine/2(Out2) -> Mux/2
  VRT_State_Machine/1(Out1) -> Mux/1
  input_time/1 -> [time]
  Voltage Command/1 -> Bus Selector1/1
  Bus Selector1/1 -> Bus Creator1/1, VRT_State_Machine/1(voltage_pha)  "<voltage_ph_a>"
  Bus Selector1/2 -> Bus Creator1/2, VRT_State_Machine/2(voltage_phb)  "<voltage_ph_b>"
  Bus Selector1/3 -> Bus Creator1/3, VRT_State_Machine/3(voltage_phc)  "<voltage_ph_c>"
  Bus Selector1/4 -> [mode]  "<mode>"
  Mux/1 -> Multiport Switch/4
  Multiport Switch/1 -> voltage_command/1
  voltage_command/1 -> voltage_magnitude_command/1
  OpWriteFile/1 -> FILE_LIMIT/1
  FILE_LIMIT/1 -> Terminator/1
  OpWriteFile/2 -> FILE_STATUS/1
  FILE_STATUS/1 -> Terminator1/1
  TRIGGER_STATUS/1 -> Terminator2/1
  Trigger_level/1 -> OpTrigger/2
  OpTrigger/1 -> TRIGGER_STATUS/1
  Mux1/1 -> OpWriteFile/1
  VRT_Trigger_End/1 -> VRT_Trigger_Start/1
  [time] -> VRT_Trigger_End/2
  Trigger High/1 -> VRT_Trigger_End/3
  VRT_Trigger/1 -> OpTrigger/1
  [time] -> VRT_Trigger_Start/2
  Trigger Low/1 -> VRT_Trigger_Start/3, VRT_Trigger_End/1
  VRT_Trigger_Start/1 -> VRT_Trigger/1
  input_meas/1 -> Mux1/1
  wavegen_mag_command/1 -> Mux1/2

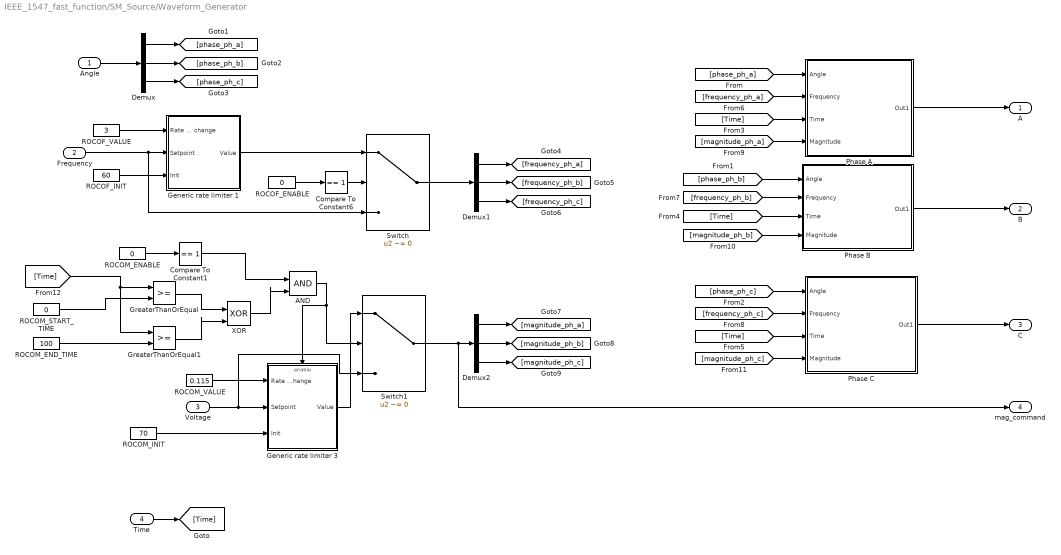
== system IEEE_1547_fast_function/SM_Source/Waveform_Generator ==
  Angle : Inport
  Frequency : Inport  Port=2
  Voltage : Inport  Port=3
  Time : Inport  Port=4
  AND : Logic  IconShape=distinctive  AllPortsSameDT=off  OutDataTypeStr=boolean
  Compare To Constant1 : simulink/Logic and Bit Operations/Compare To Constant  relop===  const=1  OutDataTypeStr=boolean
  Compare To Constant6 : simulink/Logic and Bit Operations/Compare To Constant  relop===  const=1  OutDataTypeStr=boolean
  Demux : Demux  Outputs=3
  Demux1 : Demux  Outputs=3
  Demux2 : Demux  Outputs=3
  Generic rate limiter 1 : Subsystem
  Generic rate limiter 3 : Subsystem
  GreaterThanOrEqual : RelationalOperator  OutDataTypeStr=boolean  RndMeth=Simplest
  GreaterThanOrEqual1 : RelationalOperator  OutDataTypeStr=boolean  RndMeth=Simplest
  Phase A : Subsystem
  Phase B : Subsystem
  Phase C : Subsystem
  ROCOF_ENABLE : Constant  Value=0
  ROCOF_INIT : Constant  Value=60
  ROCOF_VALUE : Constant  Value=3
  ROCOM_ENABLE : Constant  Value=0
  ROCOM_END_TIME : Constant  Value=100
  ROCOM_INIT : Constant  Value=70
  ROCOM_START_TIME : Constant  Value=0
  ROCOM_VALUE : Constant  Value=0.115
  Switch : Switch  Criteria=u2 ~= 0
  Switch1 : Switch  Criteria=u2 ~= 0
  XOR : Logic  Operator=XOR  IconShape=distinctive  AllPortsSameDT=off  OutDataTypeStr=boolean
  A : Outport
  B : Outport  Port=2
  C : Outport  Port=3
  mag_command : Outport  Port=4
  wires:
  Time/1 -> [Time]
  Phase A/1(Out1) -> A/1
  Phase B/1(Out1) -> B/1
  Phase C/1(Out1) -> C/1
  Voltage/1 -> Switch1/3, Generic rate limiter 3/2("Setpoint ")
  Angle/1 -> Demux/1
  Demux/1 -> [phase_ph_a]
  Demux/2 -> [phase_ph_b]
  Demux/3 -> [phase_ph_c]
  [phase_ph_a] -> Phase A/1(Angle)
  [phase_ph_b] -> Phase B/1(Angle)
  [phase_ph_c] -> Phase C/1(Angle)
  Generic rate limiter 1/1(Value) -> Switch/1
  Frequency/1 -> Switch/3, Generic rate limiter 1/2("Setpoint ")
  ROCOF_VALUE/1 -> Generic rate limiter 1/1(Rate of change)
  ROCOF_INIT/1 -> Generic rate limiter 1/3(Init)
  ROCOF_ENABLE/1 -> Compare To Constant6/1
  Compare To Constant6/1 -> Switch/2
  Demux1/3 -> [frequency_ph_c]
  Demux1/2 -> [frequency_ph_b]
  Demux1/1 -> [frequency_ph_a]
  Switch/1 -> Demux1/1
  ROCOM_VALUE/1 -> Generic rate limiter 3/1(Rate of change)
  ROCOM_INIT/1 -> Generic rate limiter 3/3(Init)
  [Time] -> Phase A/3(Time)
  [Time] -> Phase B/3(Time)
  [Time] -> Phase C/3(Time)
  [frequency_ph_a] -> Phase A/2(Frequency)
  [frequency_ph_b] -> Phase B/2(Frequency)
  [frequency_ph_c] -> Phase C/2(Frequency)
  Demux2/1 -> [magnitude_ph_a]
  Demux2/2 -> [magnitude_ph_b]
  Demux2/3 -> [magnitude_ph_c]
  [magnitude_ph_a] -> Phase A/4(Magnitude)
  [magnitude_ph_b] -> Phase B/4(Magnitude)
  [magnitude_ph_c] -> Phase C/4(Magnitude)
  [Time] -> GreaterThanOrEqual1/1, GreaterThanOrEqual/1
  ROCOM_START_TIME/1 -> GreaterThanOrEqual/2
  ROCOM_END_TIME/1 -> GreaterThanOrEqual1/2
  GreaterThanOrEqual/1 -> XOR/1
  GreaterThanOrEqual1/1 -> XOR/2
  Switch1/1 -> mag_command/1, Demux2/1
  Generic rate limiter 3/1(Value) -> Switch1/1
  AND/1 -> Switch1/2, Generic rate limiter 3/Enable
  XOR/1 -> AND/2
  Compare To Constant1/1 -> AND/1
  ROCOM_ENABLE/1 -> Compare To Constant1/1

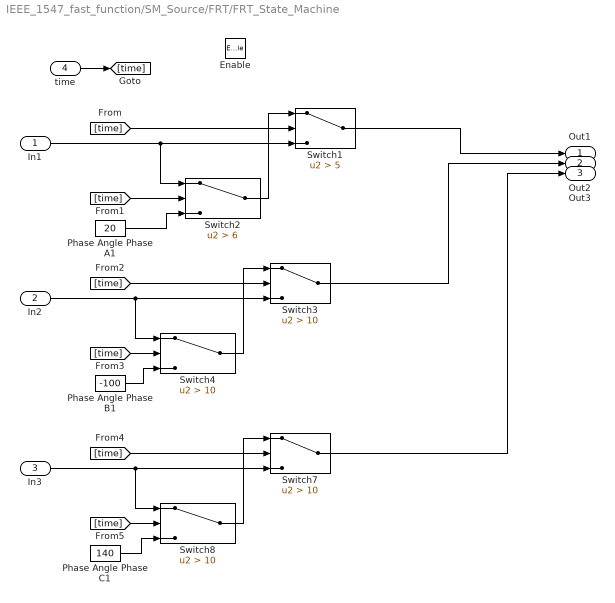
== system IEEE_1547_fast_function/SM_Source/FRT/FRT_State_Machine ==
  In1 : Inport
  In2 : Inport  Port=2
  In3 : Inport  Port=3
  time : Inport  Port=4
  Enable : EnablePort
  Phase Angle Phase A1 : Constant  Value=20
  Phase Angle Phase B1 : Constant  Value=-100
  Phase Angle Phase C1 : Constant  Value=140
  Switch1 : Switch  Criteria=u2 > Threshold  Threshold=5
  Switch2 : Switch  Criteria=u2 > Threshold  Threshold=6
  Switch{3..4,7..8} (4 alike) : Switch  Criteria=u2 > Threshold  Threshold=10
  Out1 : Outport
  Out2 : Outport  Port=2
  Out3 : Outport  Port=3
  wires:
  In3/1 -> Switch8/1, Switch7/3
  Switch2/1 -> Switch1/1
  In2/1 -> Switch4/1, Switch3/3
  Phase Angle Phase B1/1 -> Switch4/3
  Switch8/1 -> Switch7/1
  In1/1 -> Switch2/1, Switch1/3
  Switch4/1 -> Switch3/1
  Phase Angle Phase C1/1 -> Switch8/3
  Phase Angle Phase A1/1 -> Switch2/3
  [time] -> Switch8/2
  [time] -> Switch1/2
  [time] -> Switch4/2
  [time] -> Switch7/2
  [time] -> Switch2/2
  [time] -> Switch3/2
  Switch1/1 -> Out1/1
  Switch3/1 -> Out2/1
  Switch7/1 -> Out3/1
  time/1 -> [time]

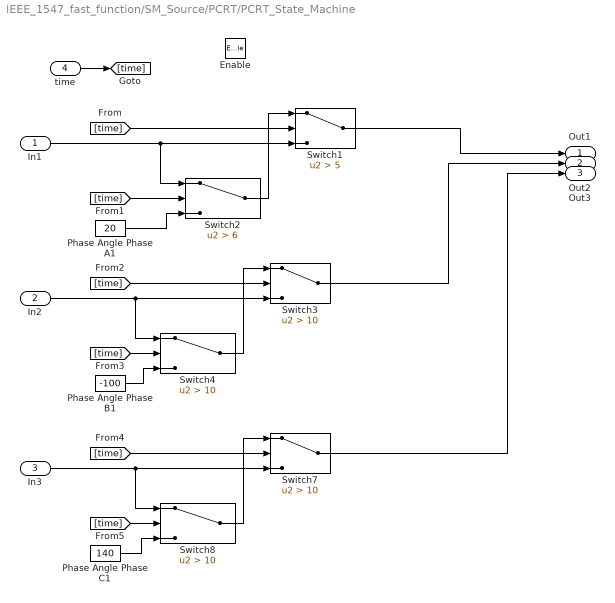
== system IEEE_1547_fast_function/SM_Source/PCRT/PCRT_State_Machine ==
  In1 : Inport
  In2 : Inport  Port=2
  In3 : Inport  Port=3
  time : Inport  Port=4
  Enable : EnablePort
  Phase Angle Phase A1 : Constant  Value=20
  Phase Angle Phase B1 : Constant  Value=-100
  Phase Angle Phase C1 : Constant  Value=140
  Switch1 : Switch  Criteria=u2 > Threshold  Threshold=5
  Switch2 : Switch  Criteria=u2 > Threshold  Threshold=6
  Switch{3..4,7..8} (4 alike) : Switch  Criteria=u2 > Threshold  Threshold=10
  Out1 : Outport
  Out2 : Outport  Port=2
  Out3 : Outport  Port=3
  wires:
  In3/1 -> Switch8/1, Switch7/3
  Switch2/1 -> Switch1/1
  In2/1 -> Switch4/1, Switch3/3
  Phase Angle Phase B1/1 -> Switch4/3
  Switch8/1 -> Switch7/1
  In1/1 -> Switch2/1, Switch1/3
  Switch4/1 -> Switch3/1
  Phase Angle Phase C1/1 -> Switch8/3
  Phase Angle Phase A1/1 -> Switch2/3
  [time] -> Switch8/2
  [time] -> Switch1/2
  [time] -> Switch4/2
  [time] -> Switch7/2
  [time] -> Switch2/2
  [time] -> Switch3/2
  Switch1/1 -> Out1/1
  Switch3/1 -> Out2/1
  Switch7/1 -> Out3/1
  time/1 -> [time]

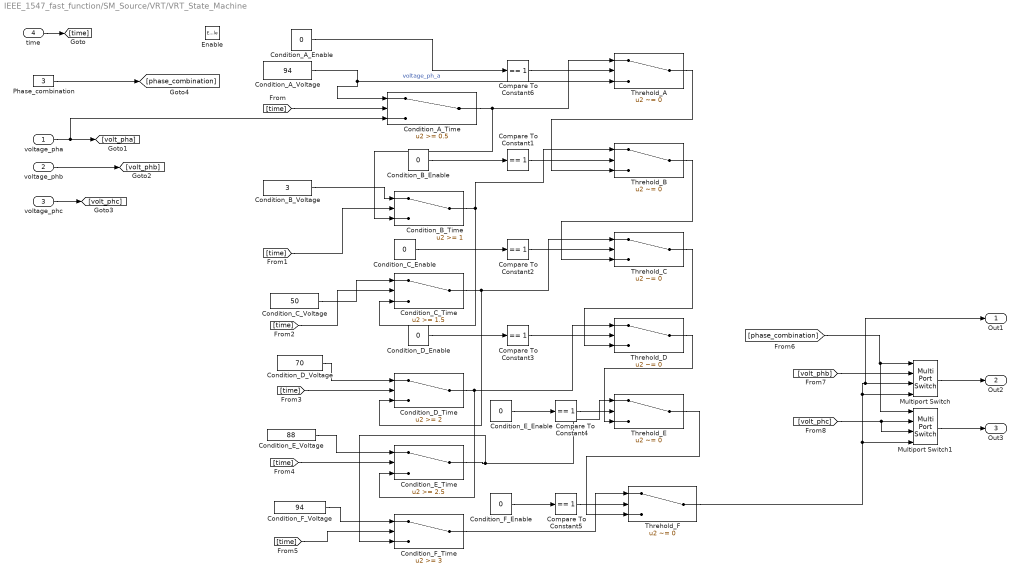
== system IEEE_1547_fast_function/SM_Source/VRT/VRT_State_Machine ==
  voltage_pha : Inport
  voltage_phb : Inport  Port=2
  voltage_phc : Inport  Port=3
  time : Inport  Port=4
  Enable : EnablePort  PropagateVarSize=During execution
  Compare To Constant{1..6} (6 alike) : simulink/Logic and Bit Operations/Compare To Constant  relop===  const=1  OutDataTypeStr=boolean
  Condition_A_Enable : Constant  Value=0
  Condition_A_Time : Switch  Threshold=0.5
  Condition_A_Voltage : Constant  Value=94
  Condition_B_Enable : Constant  Value=0
  Condition_B_Time : Switch  Threshold=1
  Condition_B_Voltage : Constant  Value=3
  Condition_C_Enable : Constant  Value=0
  Condition_C_Time : Switch  Threshold=1.5
  Condition_C_Voltage : Constant  Value=50
  Condition_D_Enable : Constant  Value=0
  Condition_D_Time : Switch  Threshold=2
  Condition_D_Voltage : Constant  Value=70
  Condition_E_Enable : Constant  Value=0
  Condition_E_Time : Switch  Threshold=2.5
  Condition_E_Voltage : Constant  Value=88
  Condition_F_Enable : Constant  Value=0
  Condition_F_Time : Switch  Threshold=3
  Condition_F_Voltage : Constant  Value=94
  Multiport Switch : MultiPortSwitch
  Multiport Switch1 : MultiPortSwitch
  Phase_combination : Constant  Value=3
  Threhold_A : Switch  Criteria=u2 ~= 0  Threshold=0.6
  Threhold_B : Switch  Criteria=u2 ~= 0  Threshold=0.6
  Threhold_C : Switch  Criteria=u2 ~= 0  Threshold=0.6
  Threhold_D : Switch  Criteria=u2 ~= 0  Threshold=0.6
  Threhold_E : Switch  Criteria=u2 ~= 0  Threshold=0.6
  Threhold_F : Switch  Criteria=u2 ~= 0  Threshold=0.6
  Out1 : Outport
  Out2 : Outport  Port=2
  Out3 : Outport  Port=3
  wires:
  time/1 -> [time]
  Phase_combination/1 -> [phase_combination]
  voltage_phb/1 -> [volt_phb]
  voltage_phc/1 -> [volt_phc]
  Multiport Switch/1 -> Out2/1
  Multiport Switch1/1 -> Out3/1
  [volt_phc] -> Multiport Switch1/3, Multiport Switch1/2
  [phase_combination] -> Multiport Switch1/1, Multiport Switch/1
  [volt_phb] -> Multiport Switch/2
  [time] -> Condition_E_Time/2
  [time] -> Condition_D_Time/2
  [time] -> Condition_F_Time/2
  [time] -> Condition_C_Time/2
  [time] -> Condition_B_Time/2
  voltage_pha/1 -> Condition_A_Time/3, [volt_pha]
  Condition_B_Voltage/1 -> Condition_B_Time/1
  Condition_C_Voltage/1 -> Condition_C_Time/1
  Condition_D_Voltage/1 -> Condition_D_Time/1
  [time] -> Condition_A_Time/2
  Condition_E_Voltage/1 -> Condition_E_Time/1
  Condition_E_Time/1 -> Condition_F_Time/3, Threhold_E/1
  Condition_A_Voltage/1 -> Condition_A_Time/1, Threhold_A/3  "voltage_ph_a"
  Condition_F_Voltage/1 -> Condition_F_Time/1
  Condition_F_Enable/1 -> Compare To Constant5/1
  Threhold_F/1 -> Out1/1, Multiport Switch/3, Multiport Switch/4, Multiport Switch1/4
  Condition_F_Time/1 -> Threhold_F/1
  Threhold_E/1 -> Threhold_F/3
  Threhold_D/1 -> Threhold_E/3
  Threhold_C/1 -> Threhold_D/3
  Threhold_B/1 -> Threhold_C/3
  Threhold_A/1 -> Threhold_B/3
  Condition_A_Time/1 -> Condition_B_Time/3, Threhold_A/1
  Condition_B_Time/1 -> Condition_C_Time/3, Threhold_B/1
  Condition_C_Time/1 -> Condition_D_Time/3, Threhold_C/1
  Condition_D_Time/1 -> Condition_E_Time/3, Threhold_D/1
  Compare To Constant6/1 -> Threhold_A/2
  Condition_B_Enable/1 -> Compare To Constant1/1
  Compare To Constant1/1 -> Threhold_B/2
  Condition_C_Enable/1 -> Compare To Constant2/1
  Compare To Constant2/1 -> Threhold_C/2
  Condition_D_Enable/1 -> Compare To Constant3/1
  Compare To Constant3/1 -> Threhold_D/2
  Condition_E_Enable/1 -> Compare To Constant4/1
  Compare To Constant4/1 -> Threhold_E/2
  Compare To Constant5/1 -> Threhold_F/2
  Condition_A_Enable/1 -> Compare To Constant6/1

== system IEEE_1547_fast_function/SM_Source/Waveform_Generator/Generic rate limiter 1 ==
  Rate of change : Inport
  "Setpoint " : Inport  Port=2
  Init : Inport  Port=3
  Add1 : Sum  Inputs=+-
  Add2 : Sum
  Gain : Gain  Gain=-1
  Rate Limiter Dynamic : simulink/Discontinuities/Rate Limiter Dynamic
      settings: SourceProductName=Simulink
  Value : Outport
  wires:
  Rate Limiter Dynamic/1 -> Add2/1  "Freq"
  Add2/1 -> Value/1  "Freq"
  Gain/1 -> Rate Limiter Dynamic/3
  Add1/1 -> Rate Limiter Dynamic/2
  "Setpoint "/1 -> Add1/1
  Rate of change/1 -> Gain/1, Rate Limiter Dynamic/1
  Init/1 -> Add1/2, Add2/2

== system IEEE_1547_fast_function/SM_Source/Waveform_Generator/Generic rate limiter 3 ==
  Rate of change : Inport
  "Setpoint " : Inport  Port=2
  Init : Inport  Port=3
  Enable : EnablePort
  Add1 : Sum  Inputs=+-
  Add2 : Sum
  Gain : Gain  Gain=-1
  Rate Limiter Dynamic : simulink/Discontinuities/Rate Limiter Dynamic
      settings: SourceProductName=Simulink
  Value : Outport
  wires:
  Init/1 -> Add2/2, Add1/2
  Rate of change/1 -> Rate Limiter Dynamic/1, Gain/1
  "Setpoint "/1 -> Add1/1
  Add1/1 -> Rate Limiter Dynamic/2
  Gain/1 -> Rate Limiter Dynamic/3
  Add2/1 -> Value/1
  Rate Limiter Dynamic/1 -> Add2/1

== system IEEE_1547_fast_function/SM_Source/Waveform_Generator/Phase A ==
  Angle : Inport
  Frequency : Inport  Port=2
  Time : Inport  Port=3
  Magnitude : Inport  Port=4
  Add2 : Sum
  Gain : Gain  Gain=2*pi
  Gain2 : Gain  Gain=pi/180
  Gain9 : Gain  Gain=sqrt(2)
  Phase A : Trigonometry
  Product2 : Product
  Product5 : Product
  Out1 : Outport
  wires:
  Angle/1 -> Gain2/1
  Phase A/1 -> Product5/1
  Gain/1 -> Product2/1
  Add2/1 -> Phase A/1
  Frequency/1 -> Gain/1
  Product2/1 -> Add2/2
  Product5/1 -> Out1/1
  Gain2/1 -> Add2/1
  Magnitude/1 -> Gain9/1
  Gain9/1 -> Product5/2
  Time/1 -> Product2/2

== system IEEE_1547_fast_function/SM_Source/Waveform_Generator/Phase B ==
  Angle : Inport
  Frequency : Inport  Port=2
  Time : Inport  Port=3
  Magnitude : Inport  Port=4
  Add2 : Sum
  Gain : Gain  Gain=2*pi
  Gain2 : Gain  Gain=pi/180
  Gain9 : Gain  Gain=sqrt(2)
  Phase A : Trigonometry
  Product2 : Product
  Product5 : Product
  Out1 : Outport
  wires:
  Time/1 -> Product2/2
  Gain9/1 -> Product5/2
  Magnitude/1 -> Gain9/1
  Gain2/1 -> Add2/1
  Product5/1 -> Out1/1
  Product2/1 -> Add2/2
  Frequency/1 -> Gain/1
  Add2/1 -> Phase A/1
  Gain/1 -> Product2/1
  Phase A/1 -> Product5/1
  Angle/1 -> Gain2/1

== system IEEE_1547_fast_function/SM_Source/Waveform_Generator/Phase C ==
  Angle : Inport
  Frequency : Inport  Port=2
  Time : Inport  Port=3
  Magnitude : Inport  Port=4
  Add2 : Sum
  Gain : Gain  Gain=2*pi
  Gain2 : Gain  Gain=pi/180
  Gain9 : Gain  Gain=sqrt(2)
  Phase A : Trigonometry
  Product2 : Product
  Product5 : Product
  Out1 : Outport
  wires:
  Angle/1 -> Gain2/1
  Phase A/1 -> Product5/1
  Gain/1 -> Product2/1
  Add2/1 -> Phase A/1
  Frequency/1 -> Gain/1
  Product2/1 -> Add2/2
  Product5/1 -> Out1/1
  Gain2/1 -> Add2/1
  Magnitude/1 -> Gain9/1
  Gain9/1 -> Product5/2
  Time/1 -> Product2/2
